simulink library "lib_Sensors"  (R2017b)
settings: Solver=VariableStepAuto  StartTime=0.0  StopTime=10.0  RelTol=1e-3
settings Model: Creator=Di Russo  LastModifiedBy=Vraj M
settings CodeAppCC: StateflowObjectComments=on

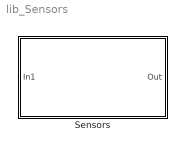
== system lib_Sensors ==
  Sensors : Subsystem

== system lib_Sensors/Sensors ==
  In1 : Inport
  Analog : Subsystem
  Bus Creator : BusCreator  Inputs=3
  Bus Selector : BusSelector  OutputSignals=CAN
  CAN : Subsystem
  Digital : Subsystem
  Out : Outport
  wires:
  Digital/1(Out1) -> Bus Creator/3  "from_Digital"
  Analog/1(Out1) -> Bus Creator/2  "from_Analog"
  CAN/1(Out1) -> Bus Creator/1  "from_CAN"
  Bus Selector/1 -> CAN/1(In1)  "<CAN>"
  In1/1 -> Bus Selector/1, Analog/1(In1), Digital/1(In1)
  Bus Creator/1 -> Out/1

== system lib_Sensors/Sensors/Analog ==
  In1 : Inport
  Bus Creator : BusCreator  Inputs=4
  Bus Selector : BusSelector  OutputSignals=Driver_Signals.drv_APP1,Driver_Signals.drv_APP2,DC_mode,Driver_Signals.Sport_Mode_SW
  Data Type Conversion : DataTypeConversion
  Data Type Conversion1 : DataTypeConversion
  Data Type Conversion2 : DataTypeConversion
  Out1 : Outport
  wires:
  Bus Selector/4 -> Bus Creator/4  "<Sport_Mode_SW>"
  Bus Selector/1 -> Data Type Conversion2/1  "<drv_APP1>"
  Bus Selector/2 -> Data Type Conversion1/1  "<drv_APP2>"
  Bus Selector/3 -> Data Type Conversion/1  "<DC_mode>"
  Bus Creator/1 -> Out1/1
  In1/1 -> Bus Selector/1
  Data Type Conversion2/1 -> Bus Creator/1  "Driver_APP1"
  Data Type Conversion1/1 -> Bus Creator/2  "Driver_APP2"
  Data Type Conversion/1 -> Bus Creator/3  "DC_mode"

== system lib_Sensors/Sensors/CAN ==
  In1 : Inport
  Bus Creator : BusCreator  Inputs=3
  EBCAN : Subsystem
  HV_CAN : Subsystem
  VEH_CAN : Subsystem
  Out1 : Outport
  wires:
  VEH_CAN/1(Out1) -> Bus Creator/1  "fromVEH_CAN"
  Bus Creator/1 -> Out1/1  "from_CAN"
  EBCAN/1(Out1) -> Bus Creator/2  "fromEBCAN"
  HV_CAN/1(Out1) -> Bus Creator/3  "fromHV_CAN"
  In1/1 -> HV_CAN/1(In1), EBCAN/1(In1), VEH_CAN/1(In1)

== system lib_Sensors/Sensors/Digital ==
  In1 : Inport
  Bus Creator : BusCreator  Inputs=3
  Bus Selector : BusSelector  OutputSignals=Driver_Signals.SW_Regen_Disable,Driver_Signals.SW_Engine_ON,Driver_Signals.SW_CS_ON
  Data Type Conversion : DataTypeConversion
  Data Type Conversion1 : DataTypeConversion
  Data Type Conversion2 : DataTypeConversion
  Out1 : Outport
  wires:
  Bus Creator/1 -> Out1/1  "Digital"
  Data Type Conversion1/1 -> Bus Creator/1  "SW_Regen_Disable"
  Data Type Conversion2/1 -> Bus Creator/3  "SW_CS_ON"
  Data Type Conversion/1 -> Bus Creator/2  "SW_Engine_ON"
  Bus Selector/3 -> Data Type Conversion2/1  "<SW_CS_ON>"
  Bus Selector/2 -> Data Type Conversion/1  "<SW_Engine_ON>"
  Bus Selector/1 -> Data Type Conversion1/1  "<SW_Regen_Disable>"
  In1/1 -> Bus Selector/1

== system lib_Sensors/Sensors/CAN/EBCAN ==
  In1 : Inport
  BMS_Antrieb : Subsystem
  Bus Creator : BusCreator  Inputs=3
  Bus Selector : BusSelector  OutputSignals=ECM_CAN,BMS_CAN.BMS_Hybrid
  CCM : Subsystem
  ECM : Subsystem
  Out1 : Outport
  wires:
  ECM/1(Out1) -> Bus Creator/1  "from_ECM"
  BMS_Antrieb/1(Out1) -> Bus Creator/2  "from_BMSAntrieb"
  Bus Creator/1 -> Out1/1
  CCM/1(Out1) -> Bus Creator/3  "from_CCM"
  In1/1 -> Bus Selector/1
  Bus Selector/1 -> ECM/1(In1)  "<ECM_CAN>"
  Bus Selector/2 -> CCM/1(In1), BMS_Antrieb/1(In1)  "<BMS_Hybrid>"

== system lib_Sensors/Sensors/CAN/HV_CAN ==
  In1 : Inport
  BMS_Hybrid : Subsystem
  Bus Creator : BusCreator  Inputs=4
  Bus Selector : BusSelector  OutputSignals=MCU_CAN,BMS_CAN.BMS_Plugin,OBC_CAN
  Clutch : Subsystem
  MCU : Subsystem
  OBC : Subsystem
  Out1 : Outport
  wires:
  MCU/1(Out1) -> Bus Creator/2  "from_MCU"
  BMS_Hybrid/1(Out1) -> Bus Creator/3  "from_BMSHybrid"
  OBC/1(Out1) -> Bus Creator/4  "from_OBC"
  Bus Creator/1 -> Out1/1
  In1/1 -> Bus Selector/1
  Bus Selector/1 -> Clutch/1(In1), MCU/1(In1)  "<MCU_CAN>"
  Bus Selector/2 -> BMS_Hybrid/1(In1)  "<BMS_Plugin>"
  Bus Selector/3 -> OBC/1(In1)  "<OBC_CAN>"
  Clutch/1(Out1) -> Bus Creator/1

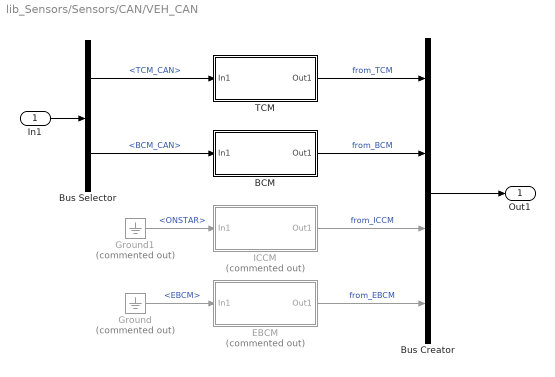
== system lib_Sensors/Sensors/CAN/VEH_CAN ==
  In1 : Inport
  BCM : Subsystem
  Bus Creator : BusCreator  Inputs=4
  Bus Selector : BusSelector  OutputSignals=TCM_CAN,BCM_CAN
  EBCM : Subsystem  Commented=on
  Ground : Ground  Commented=on
  Ground1 : Ground  Commented=on
  ICCM : Subsystem  Commented=on
  TCM : Subsystem
  Out1 : Outport
  wires:
  In1/1 -> Bus Selector/1
  TCM/1(Out1) -> Bus Creator/1  "from_TCM"
  BCM/1(Out1) -> Bus Creator/2  "from_BCM"
  ICCM/1(Out1) -> Bus Creator/3  "from_ICCM"
  EBCM/1(Out1) -> Bus Creator/4  "from_EBCM"
  Bus Creator/1 -> Out1/1
  Bus Selector/1 -> TCM/1(In1)  "<TCM_CAN>"
  Bus Selector/2 -> BCM/1(In1)  "<BCM_CAN>"
  Ground1/1 -> ICCM/1(In1)  "<ONSTAR>"
  Ground/1 -> EBCM/1(In1)  "<EBCM>"

== system lib_Sensors/Sensors/CAN/EBCAN/BMS_Antrieb ==
  In1 : Inport
  Bus Creator : BusCreator  Inputs=2
  Bus Selector : BusSelector  OutputSignals=NMH_BMS,ISO_Hybrid_01_Resp
  ISO_Hybrid_01_Resp : Subsystem
  NMH_BMS : Subsystem
  Out1 : Outport
  wires:
  In1/1 -> Bus Selector/1
  Bus Selector/1 -> NMH_BMS/1(In1)  "<NMH_BMS>"
  NMH_BMS/1(Out1) -> Bus Creator/1
  ISO_Hybrid_01_Resp/1(Out1) -> Bus Creator/2
  Bus Creator/1 -> Out1/1
  Bus Selector/2 -> ISO_Hybrid_01_Resp/1(In1)  "<ISO_Hybrid_01_Resp>"

== system lib_Sensors/Sensors/CAN/EBCAN/CCM ==
  In1 : Inport
  Bus Creator : BusCreator  Inputs=2
  Bus Selector : BusSelector  OutputSignals=NMH_BMS,ISO_Hybrid_01_Resp
  ISO_Hybrid_01_Resp : Subsystem
  NMH_BMS : Subsystem
  Out1 : Outport
  wires:
  Bus Selector/2 -> ISO_Hybrid_01_Resp/1(In1)  "<ISO_Hybrid_01_Resp>"
  Bus Creator/1 -> Out1/1
  ISO_Hybrid_01_Resp/1(Out1) -> Bus Creator/2
  NMH_BMS/1(Out1) -> Bus Creator/1
  Bus Selector/1 -> NMH_BMS/1(In1)  "<NMH_BMS>"
  In1/1 -> Bus Selector/1

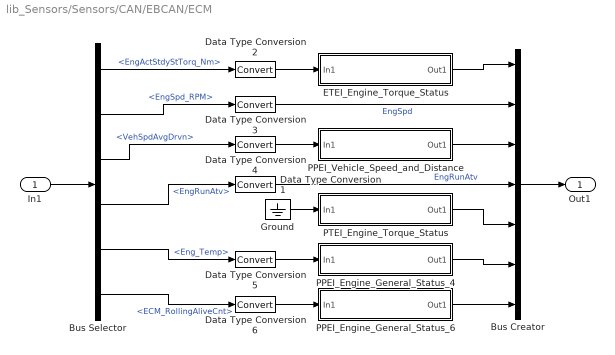
== system lib_Sensors/Sensors/CAN/EBCAN/ECM ==
  In1 : Inport
  Bus Creator : BusCreator  Inputs=7
  Bus Selector : BusSelector  OutputSignals=Sensors_to_ECM.EngActStdyStTorq_Nm,Sensors_to_ECM.EngSpd_RPM,ECM_to_Actuators.VehSpdAvgDrvn,ECM_to_Actuators.EngRunAtv,ECM_to_Actuators.Eng_Temp,ECM_to_Actuators.ECM_RollingAliveCnt
  Data Type Conversion{1..6} (6 alike) : DataTypeConversion
  ETEI_Engine_Torque_Status : Subsystem
  Ground : Ground
  PPEI_Engine_General_Status_4 : Subsystem
  PPEI_Engine_General_Status_6 : Subsystem
  PPEI_Vehicle_Speed_and_Distance : Subsystem
  PTEI_Engine_Torque_Status : Subsystem
  Out1 : Outport
  wires:
  Bus Selector/6 -> Data Type Conversion6/1  "<ECM_RollingAliveCnt>"
  Bus Selector/5 -> Data Type Conversion5/1  "<Eng_Temp>"
  Bus Selector/3 -> Data Type Conversion4/1  "<VehSpdAvgDrvn>"
  Bus Selector/1 -> Data Type Conversion2/1  "<EngActStdyStTorq_Nm>"
  In1/1 -> Bus Selector/1
  Data Type Conversion2/1 -> ETEI_Engine_Torque_Status/1(In1)
  Bus Selector/2 -> Data Type Conversion3/1  "<EngSpd_RPM>"
  Data Type Conversion4/1 -> PPEI_Vehicle_Speed_and_Distance/1(In1)
  ETEI_Engine_Torque_Status/1(Out1) -> Bus Creator/1
  PPEI_Vehicle_Speed_and_Distance/1(Out1) -> Bus Creator/3
  Bus Creator/1 -> Out1/1
  Bus Selector/4 -> Data Type Conversion1/1  "<EngRunAtv>"
  Ground/1 -> PTEI_Engine_Torque_Status/1(In1)
  PTEI_Engine_Torque_Status/1(Out1) -> Bus Creator/5
  Data Type Conversion5/1 -> PPEI_Engine_General_Status_4/1(In1)
  PPEI_Engine_General_Status_4/1(Out1) -> Bus Creator/6
  Data Type Conversion6/1 -> PPEI_Engine_General_Status_6/1(In1)
  PPEI_Engine_General_Status_6/1(Out1) -> Bus Creator/7
  Data Type Conversion3/1 -> Bus Creator/2  "EngSpd"
  Data Type Conversion1/1 -> Bus Creator/4  "EngRunAtv"

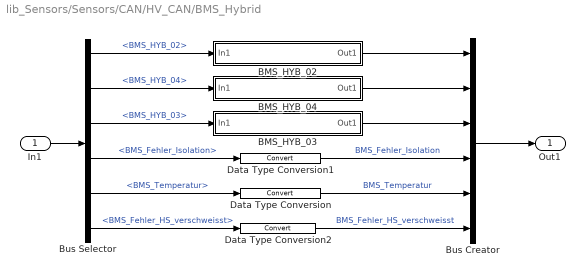
== system lib_Sensors/Sensors/CAN/HV_CAN/BMS_Hybrid ==
  In1 : Inport
  BMS_HYB_02 : Subsystem
  BMS_HYB_03 : Subsystem
  BMS_HYB_04 : Subsystem
  Bus Creator : BusCreator  Inputs=6
  Bus Selector : BusSelector  OutputSignals=BMS_HYB_02,BMS_HYB_04,BMS_HYB_03,BMS_HYB_02.BMS_Fehler_Isolation,BMS_HYB_06.BMS_Temperatur,BMS_HYB_02.BMS_Fehler_HS_verschweisst
  Data Type Conversion : DataTypeConversion
  Data Type Conversion1 : DataTypeConversion
  Data Type Conversion2 : DataTypeConversion
  Out1 : Outport
  wires:
  Bus Selector/6 -> Data Type Conversion2/1  "<BMS_Fehler_HS_verschweisst>"
  Data Type Conversion1/1 -> Bus Creator/4  "BMS_Fehler_Isolation"
  Data Type Conversion/1 -> Bus Creator/5  "BMS_Temperatur"
  In1/1 -> Bus Selector/1
  Bus Selector/1 -> BMS_HYB_02/1(In1)  "<BMS_HYB_02>"
  Bus Selector/2 -> BMS_HYB_04/1(In1)  "<BMS_HYB_04>"
  Bus Creator/1 -> Out1/1
  BMS_HYB_02/1(Out1) -> Bus Creator/1
  BMS_HYB_04/1(Out1) -> Bus Creator/2
  Bus Selector/3 -> BMS_HYB_03/1(In1)  "<BMS_HYB_03>"
  BMS_HYB_03/1(Out1) -> Bus Creator/3
  Bus Selector/4 -> Data Type Conversion1/1  "<BMS_Fehler_Isolation>"
  Bus Selector/5 -> Data Type Conversion/1  "<BMS_Temperatur>"
  Data Type Conversion2/1 -> Bus Creator/6  "BMS_Fehler_HS_verschweisst"

== system lib_Sensors/Sensors/CAN/HV_CAN/Clutch ==
  In1 : Inport
  Bus Creator : BusCreator  Inputs=2
  Bus Selector : BusSelector  OutputSignals=MCU_to _Actuator.EngageClutch,Sensors_to_MCU.clt_plant_spd_in
  Data Type Conversion : DataTypeConversion
  Data Type Conversion1 : DataTypeConversion
  Out1 : Outport
  wires:
  Bus Selector/2 -> Data Type Conversion1/1  "<clt_plant_spd_in>"
  Data Type Conversion1/1 -> Bus Creator/2  "CY01_AngSpdCurr"
  Data Type Conversion/1 -> Bus Creator/1  "CY01_posCurr"
  Bus Selector/1 -> Data Type Conversion/1  "<EngageClutch>"
  Bus Creator/1 -> Out1/1  "Clutch"
  In1/1 -> Bus Selector/1

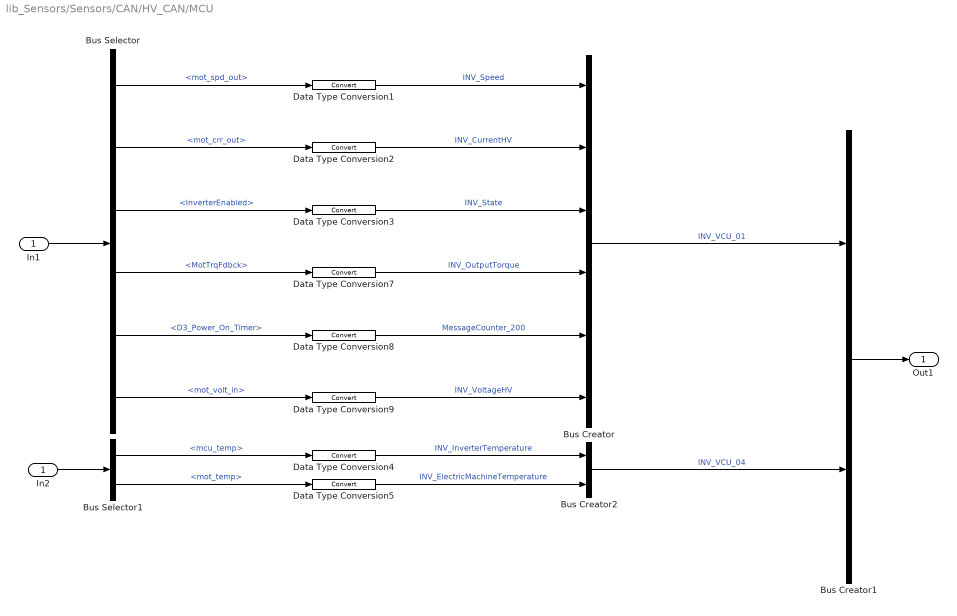
== system lib_Sensors/Sensors/CAN/HV_CAN/MCU ==
  In1 : Inport
  Bus Creator : BusCreator  Inputs=6
  Bus Creator1 : BusCreator  Inputs=2
  Bus Creator2 : BusCreator  Inputs=2
  Bus Selector : BusSelector  OutputSignals=Sensors_to_MCU.mot_spd_out,Sensors_to_MCU.mot_crr_out,MCU_to _Actuator.InverterEnabled,MCU_to _Actuator.MotTrqFdbck,MCU_to _Actuator.D3_Power_On_Timer,Sensors_to_MCU.mot_volt_in
  Bus Selector1 : BusSelector  OutputSignals=Sensors_to_MCU.mcu_temp,Sensors_to_MCU.mot_temp
  Data Type Conversion{1..5,7..9} (8 alike) : DataTypeConversion
  In2 : InportShadow
  Out1 : Outport
  wires:
  Bus Creator1/1 -> Out1/1
  Bus Creator2/1 -> Bus Creator1/2  "INV_VCU_04"
  In2/1 -> Bus Selector1/1
  Bus Selector1/1 -> Data Type Conversion4/1  "<mcu_temp>"
  Data Type Conversion5/1 -> Bus Creator2/2  "INV_ElectricMachineTemperature"
  Bus Selector1/2 -> Data Type Conversion5/1  "<mot_temp>"
  Data Type Conversion4/1 -> Bus Creator2/1  "INV_InverterTemperature"
  Data Type Conversion9/1 -> Bus Creator/6  "INV_VoltageHV"
  Data Type Conversion8/1 -> Bus Creator/5  "MessageCounter_200"
  Data Type Conversion7/1 -> Bus Creator/4  "INV_OutputTorque"
  Bus Selector/1 -> Data Type Conversion1/1  "<mot_spd_out>"
  Bus Selector/2 -> Data Type Conversion2/1  "<mot_crr_out>"
  Bus Selector/3 -> Data Type Conversion3/1  "<InverterEnabled>"
  Data Type Conversion1/1 -> Bus Creator/1  "INV_Speed"
  Data Type Conversion2/1 -> Bus Creator/2  "INV_CurrentHV"
  Data Type Conversion3/1 -> Bus Creator/3  "INV_State"
  Bus Creator/1 -> Bus Creator1/1  "INV_VCU_01"
  Bus Selector/5 -> Data Type Conversion8/1  "<D3_Power_On_Timer>"
  Bus Selector/4 -> Data Type Conversion7/1  "<MotTrqFdbck>"
  Bus Selector/6 -> Data Type Conversion9/1  "<mot_volt_in>"
  In1/1 -> Bus Selector/1

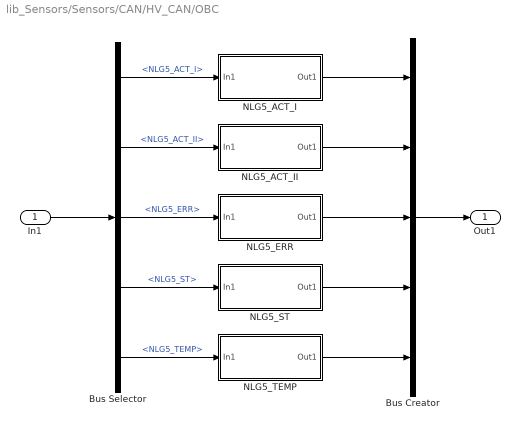
== system lib_Sensors/Sensors/CAN/HV_CAN/OBC ==
  In1 : Inport
  Bus Creator : BusCreator  Inputs=5
  Bus Selector : BusSelector  OutputSignals=NLG5_ACT_I,NLG5_ACT_II,NLG5_ERR,NLG5_ST,NLG5_TEMP
  NLG5_ACT_I : Subsystem
  NLG5_ACT_II : Subsystem
  NLG5_ERR : Subsystem
  NLG5_ST : Subsystem
  NLG5_TEMP : Subsystem
  Out1 : Outport
  wires:
  Bus Creator/1 -> Out1/1
  NLG5_TEMP/1(Out1) -> Bus Creator/5
  Bus Selector/5 -> NLG5_TEMP/1(In1)  "<NLG5_TEMP>"
  NLG5_ST/1(Out1) -> Bus Creator/4
  Bus Selector/4 -> NLG5_ST/1(In1)  "<NLG5_ST>"
  Bus Selector/3 -> NLG5_ERR/1(In1)  "<NLG5_ERR>"
  NLG5_ERR/1(Out1) -> Bus Creator/3
  NLG5_ACT_II/1(Out1) -> Bus Creator/2
  Bus Selector/2 -> NLG5_ACT_II/1(In1)  "<NLG5_ACT_II>"
  NLG5_ACT_I/1(Out1) -> Bus Creator/1
  Bus Selector/1 -> NLG5_ACT_I/1(In1)  "<NLG5_ACT_I>"
  In1/1 -> Bus Selector/1

== system lib_Sensors/Sensors/CAN/VEH_CAN/BCM ==
  In1 : Inport
  Bus Creator : BusCreator  Inputs=2
  Bus Selector : BusSelector  OutputSignals=SysPwrMd,BrkPdlPos
  Data Type Conversion : DataTypeConversion
  Data Type Conversion1 : DataTypeConversion
  PPEI_Brake_Apply_Status : Subsystem
  PPEI_Platfrom_General_Status : Subsystem
  Out1 : Outport
  wires:
  In1/1 -> Bus Selector/1
  Bus Selector/1 -> Data Type Conversion/1  "<SysPwrMd>"
  Bus Selector/2 -> Data Type Conversion1/1  "<BrkPdlPos>"
  PPEI_Platfrom_General_Status/1(Out1) -> Bus Creator/1
  PPEI_Brake_Apply_Status/1(Out1) -> Bus Creator/2
  Bus Creator/1 -> Out1/1
  Data Type Conversion/1 -> PPEI_Platfrom_General_Status/1(In1)
  Data Type Conversion1/1 -> PPEI_Brake_Apply_Status/1(In1)

== system lib_Sensors/Sensors/CAN/VEH_CAN/EBCM ==
  In1 : Inport
  Bus Selector : BusSelector  OutputSignals=PPEI_Chassis_General_Status_1.BrkPdlDrvAppPrsDetcd
  Constant : Constant  OutDataTypeStr=boolean
  PPEI_Chassis_General_Status_1 : Subsystem
  Terminator : Terminator
  Out1 : Outport
  wires:
  Bus Selector/1 -> Terminator/1  "<BrkPdlDrvAppPrsDetcd>"
  PPEI_Chassis_General_Status_1/1(Out1) -> Out1/1
  In1/1 -> Bus Selector/1
  Constant/1 -> PPEI_Chassis_General_Status_1/1(In1)

== system lib_Sensors/Sensors/CAN/VEH_CAN/ICCM ==
  In1 : Inport
  Out1 : Outport
  wires:
  In1/1 -> Out1/1

== system lib_Sensors/Sensors/CAN/VEH_CAN/TCM ==
  In1 : Inport
  Bus Creator : BusCreator  Inputs=4
  Bus Selector : BusSelector  OutputSignals=TCM_to _Actuator.TransEstGear,TCM_to _Actuator.LockupCmd,TCM_to _Actuator.TrnsShftLvrPos,Sensors_to_TCM.gb_trq_ratio
  Data Type Conversion{,1..3} (4 alike) : DataTypeConversion
  Out1 : Outport
  wires:
  Bus Selector/4 -> Data Type Conversion3/1  "<gb_trq_ratio>"
  Bus Selector/3 -> Data Type Conversion2/1  "<TrnsShftLvrPos>"
  Bus Selector/2 -> Data Type Conversion1/1  "<LockupCmd>"
  Bus Selector/1 -> Data Type Conversion/1  "<TransEstGear>"
  Data Type Conversion3/1 -> Bus Creator/4  "TrnGrRat"
  Data Type Conversion2/1 -> Bus Creator/3  "TrnsShftLvrPos"
  Data Type Conversion1/1 -> Bus Creator/2  "TrnsTrqCnvCltCmndMd"
  In1/1 -> Bus Selector/1
  Bus Creator/1 -> Out1/1
  Data Type Conversion/1 -> Bus Creator/1  "TransEstGear"

== system lib_Sensors/Sensors/CAN/EBCAN/BMS_Antrieb/ISO_Hybrid_01_Resp ==
  In1 : Inport
  Bus Creator : BusCreator  Inputs=3
  Bus Selector : BusSelector  OutputSignals=ISO_Hybrid_01_Resp_Data_4,ISO_Hybrid_01_Resp_Data_5,ISO_Hybrid_01_Resp_Data_6
  Data Type Conversion : DataTypeConversion
  Data Type Conversion1 : DataTypeConversion
  Data Type Conversion2 : DataTypeConversion
  Out1 : Outport
  wires:
  Data Type Conversion2/1 -> Bus Creator/3  "ISO_Hybrid_01_Resp_Data_byte_5"
  Data Type Conversion1/1 -> Bus Creator/2  "ISO_Hybrid_01_Resp_Data_byte_4"
  Data Type Conversion/1 -> Bus Creator/1  "ISO_Hybrid_01_Resp_Data_byte_3"
  Bus Creator/1 -> Out1/1  "ISO_Hybrid_01_Resp_Data"
  Bus Selector/3 -> Data Type Conversion2/1  "<ISO_Hybrid_01_Resp_Data_6>"
  Bus Selector/2 -> Data Type Conversion1/1  "<ISO_Hybrid_01_Resp_Data_5>"
  Bus Selector/1 -> Data Type Conversion/1  "<ISO_Hybrid_01_Resp_Data_4>"
  In1/1 -> Bus Selector/1

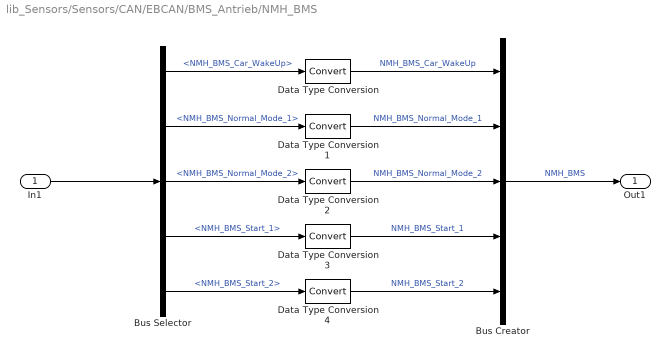
== system lib_Sensors/Sensors/CAN/EBCAN/BMS_Antrieb/NMH_BMS ==
  In1 : Inport
  Bus Creator : BusCreator  Inputs=5
  Bus Selector : BusSelector  OutputSignals=NMH_BMS_Car_WakeUp,NMH_BMS_Normal_Mode_1,NMH_BMS_Normal_Mode_2,NMH_BMS_Start_1,NMH_BMS_Start_2
  Data Type Conversion{,1..4} (5 alike) : DataTypeConversion
  Out1 : Outport
  wires:
  Data Type Conversion4/1 -> Bus Creator/5  "NMH_BMS_Start_2"
  Data Type Conversion3/1 -> Bus Creator/4  "NMH_BMS_Start_1"
  Data Type Conversion2/1 -> Bus Creator/3  "NMH_BMS_Normal_Mode_2"
  Data Type Conversion1/1 -> Bus Creator/2  "NMH_BMS_Normal_Mode_1"
  Data Type Conversion/1 -> Bus Creator/1  "NMH_BMS_Car_WakeUp"
  Bus Selector/1 -> Data Type Conversion/1  "<NMH_BMS_Car_WakeUp>"
  Bus Selector/2 -> Data Type Conversion1/1  "<NMH_BMS_Normal_Mode_1>"
  Bus Selector/3 -> Data Type Conversion2/1  "<NMH_BMS_Normal_Mode_2>"
  Bus Selector/4 -> Data Type Conversion3/1  "<NMH_BMS_Start_1>"
  Bus Selector/5 -> Data Type Conversion4/1  "<NMH_BMS_Start_2>"
  Bus Creator/1 -> Out1/1  "NMH_BMS"
  In1/1 -> Bus Selector/1

== system lib_Sensors/Sensors/CAN/EBCAN/CCM/ISO_Hybrid_01_Resp ==
  In1 : Inport
  Bus Creator : BusCreator  Inputs=3
  Bus Selector : BusSelector  OutputSignals=ISO_Hybrid_01_Resp_Data_4,ISO_Hybrid_01_Resp_Data_5,ISO_Hybrid_01_Resp_Data_6
  Data Type Conversion : DataTypeConversion
  Data Type Conversion1 : DataTypeConversion
  Data Type Conversion2 : DataTypeConversion
  Out1 : Outport
  wires:
  In1/1 -> Bus Selector/1
  Bus Selector/1 -> Data Type Conversion/1  "<ISO_Hybrid_01_Resp_Data_4>"
  Bus Selector/2 -> Data Type Conversion1/1  "<ISO_Hybrid_01_Resp_Data_5>"
  Bus Selector/3 -> Data Type Conversion2/1  "<ISO_Hybrid_01_Resp_Data_6>"
  Bus Creator/1 -> Out1/1  "ISO_Hybrid_01_Resp_Data"
  Data Type Conversion/1 -> Bus Creator/1  "ISO_Hybrid_01_Resp_Data_byte_3"
  Data Type Conversion1/1 -> Bus Creator/2  "ISO_Hybrid_01_Resp_Data_byte_4"
  Data Type Conversion2/1 -> Bus Creator/3  "ISO_Hybrid_01_Resp_Data_byte_5"

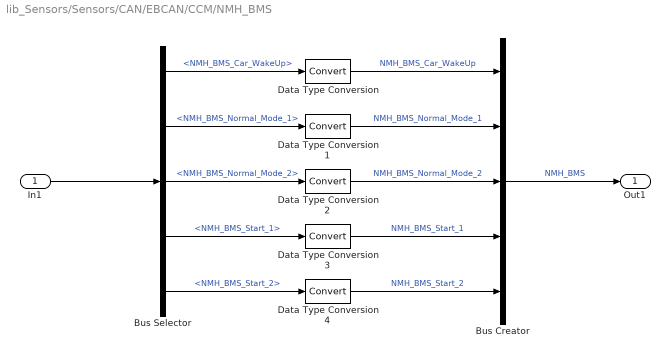
== system lib_Sensors/Sensors/CAN/EBCAN/CCM/NMH_BMS ==
  In1 : Inport
  Bus Creator : BusCreator  Inputs=5
  Bus Selector : BusSelector  OutputSignals=NMH_BMS_Car_WakeUp,NMH_BMS_Normal_Mode_1,NMH_BMS_Normal_Mode_2,NMH_BMS_Start_1,NMH_BMS_Start_2
  Data Type Conversion{,1..4} (5 alike) : DataTypeConversion
  Out1 : Outport
  wires:
  In1/1 -> Bus Selector/1
  Bus Creator/1 -> Out1/1  "NMH_BMS"
  Bus Selector/5 -> Data Type Conversion4/1  "<NMH_BMS_Start_2>"
  Bus Selector/4 -> Data Type Conversion3/1  "<NMH_BMS_Start_1>"
  Bus Selector/3 -> Data Type Conversion2/1  "<NMH_BMS_Normal_Mode_2>"
  Bus Selector/2 -> Data Type Conversion1/1  "<NMH_BMS_Normal_Mode_1>"
  Bus Selector/1 -> Data Type Conversion/1  "<NMH_BMS_Car_WakeUp>"
  Data Type Conversion/1 -> Bus Creator/1  "NMH_BMS_Car_WakeUp"
  Data Type Conversion1/1 -> Bus Creator/2  "NMH_BMS_Normal_Mode_1"
  Data Type Conversion2/1 -> Bus Creator/3  "NMH_BMS_Normal_Mode_2"
  Data Type Conversion3/1 -> Bus Creator/4  "NMH_BMS_Start_1"
  Data Type Conversion4/1 -> Bus Creator/5  "NMH_BMS_Start_2"

== system lib_Sensors/Sensors/CAN/EBCAN/ECM/ETEI_Engine_Torque_Status ==
  In1 : Inport
  Out1 : Outport
  wires:
  In1/1 -> Out1/1  "EngActStdyStTorq"

== system lib_Sensors/Sensors/CAN/EBCAN/ECM/PPEI_Engine_General_Status_4 ==
  In1 : Inport
  Out1 : Outport
  wires:
  In1/1 -> Out1/1  "EngCltTmp"

== system lib_Sensors/Sensors/CAN/EBCAN/ECM/PPEI_Engine_General_Status_6 ==
  In1 : Inport
  Out1 : Outport
  wires:
  In1/1 -> Out1/1  "PlatEngSpdCmdStARC"

== system lib_Sensors/Sensors/CAN/EBCAN/ECM/PPEI_Vehicle_Speed_and_Distance ==
  In1 : Inport
  Out1 : Outport
  wires:
  In1/1 -> Out1/1  "VehSpdAvgDrvn"

== system lib_Sensors/Sensors/CAN/EBCAN/ECM/PTEI_Engine_Torque_Status ==
  In1 : Inport
  Out1 : Outport
  wires:
  In1/1 -> Out1/1  "CrksftNTrnsRegCmdTq"

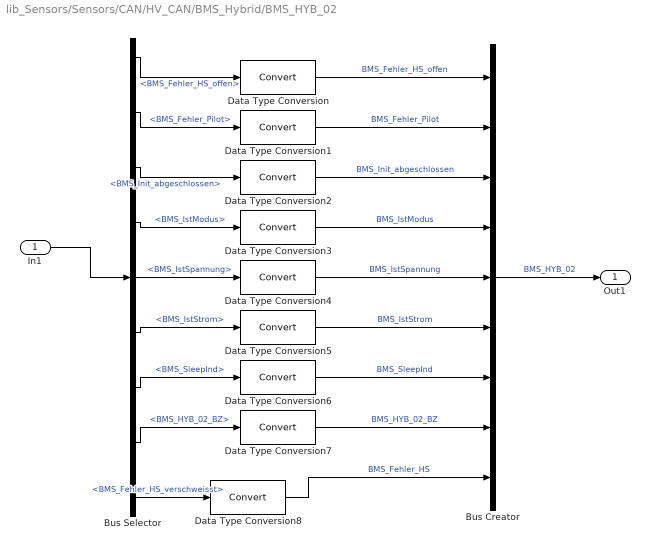
== system lib_Sensors/Sensors/CAN/HV_CAN/BMS_Hybrid/BMS_HYB_02 ==
  In1 : Inport
  Bus Creator : BusCreator  Inputs=9
  Bus Selector : BusSelector  OutputSignals=BMS_Fehler_HS_offen,BMS_Fehler_Pilot,BMS_Init_abgeschlossen,BMS_IstModus,BMS_IstSpannung,BMS_IstStrom,BMS_SleepInd,BMS_HYB_02_BZ,BMS_Fehler_HS_verschweisst
  Data Type Conversion{,1..8} (9 alike) : DataTypeConversion
  Out1 : Outport
  wires:
  Data Type Conversion8/1 -> Bus Creator/9  "BMS_Fehler_HS"
  Data Type Conversion7/1 -> Bus Creator/8  "BMS_HYB_02_BZ"
  Data Type Conversion6/1 -> Bus Creator/7  "BMS_SleepInd"
  Data Type Conversion5/1 -> Bus Creator/6  "BMS_IstStrom"
  Data Type Conversion4/1 -> Bus Creator/5  "BMS_IstSpannung"
  Data Type Conversion3/1 -> Bus Creator/4  "BMS_IstModus"
  Data Type Conversion2/1 -> Bus Creator/3  "BMS_Init_abgeschlossen"
  Data Type Conversion1/1 -> Bus Creator/2  "BMS_Fehler_Pilot"
  Data Type Conversion/1 -> Bus Creator/1  "BMS_Fehler_HS_offen"
  Bus Selector/1 -> Data Type Conversion/1  "<BMS_Fehler_HS_offen>"
  Bus Selector/2 -> Data Type Conversion1/1  "<BMS_Fehler_Pilot>"
  Bus Selector/3 -> Data Type Conversion2/1  "<BMS_Init_abgeschlossen>"
  Bus Selector/4 -> Data Type Conversion3/1  "<BMS_IstModus>"
  Bus Selector/5 -> Data Type Conversion4/1  "<BMS_IstSpannung>"
  Bus Selector/6 -> Data Type Conversion5/1  "<BMS_IstStrom>"
  Bus Selector/7 -> Data Type Conversion6/1  "<BMS_SleepInd>"
  Bus Creator/1 -> Out1/1  "BMS_HYB_02"
  In1/1 -> Bus Selector/1
  Bus Selector/8 -> Data Type Conversion7/1  "<BMS_HYB_02_BZ>"
  Bus Selector/9 -> Data Type Conversion8/1  "<BMS_Fehler_HS_verschweisst>"

== system lib_Sensors/Sensors/CAN/HV_CAN/BMS_Hybrid/BMS_HYB_03 ==
  In1 : Inport
  Bus Selector : BusSelector  OutputSignals=BMS_SOC
  Data Type Conversion : DataTypeConversion
  Out1 : Outport
  wires:
  Data Type Conversion/1 -> Out1/1  "BMS_SOC"
  Bus Selector/1 -> Data Type Conversion/1  "<BMS_SOC>"
  In1/1 -> Bus Selector/1

== system lib_Sensors/Sensors/CAN/HV_CAN/BMS_Hybrid/BMS_HYB_04 ==
  In1 : Inport
  Bus Selector : BusSelector  OutputSignals=BMS_Spannung_ZwKr
  Data Type Conversion : DataTypeConversion
  Out1 : Outport
  wires:
  Data Type Conversion/1 -> Out1/1  "BMS_Spannung_ZwKr"
  In1/1 -> Bus Selector/1  "BMS_Spannung_ZwKr"
  Bus Selector/1 -> Data Type Conversion/1  "<BMS_Spannung_ZwKr>"

== system lib_Sensors/Sensors/CAN/HV_CAN/OBC/NLG5_ACT_I ==
  In1 : Inport
  Bus Creator : BusCreator  Inputs=4
  Bus Selector : BusSelector  OutputSignals=signal1,NLG5_MV_ACT,NLG5_OV_ACT,NLG5_OC_ACT
  Data Type Conversion{,1..3} (4 alike) : DataTypeConversion
  Out1 : Outport
  wires:
  Bus Creator/1 -> Out1/1  "NLG5_ACT_I"
  Data Type Conversion3/1 -> Bus Creator/4  "NLG5_OC_ACT"
  Data Type Conversion2/1 -> Bus Creator/3  "NLG5_OV_ACT"
  Data Type Conversion1/1 -> Bus Creator/2  "NLG5_MV_ACT"
  Data Type Conversion/1 -> Bus Creator/1  "NLG5_MC_ACT"
  Bus Selector/4 -> Data Type Conversion3/1  "<NLG5_OC_ACT>"
  Bus Selector/3 -> Data Type Conversion2/1  "<NLG5_OV_ACT>"
  Bus Selector/2 -> Data Type Conversion1/1  "<NLG5_MV_ACT>"
  Bus Selector/1 -> Data Type Conversion/1  "<signal1>"
  In1/1 -> Bus Selector/1

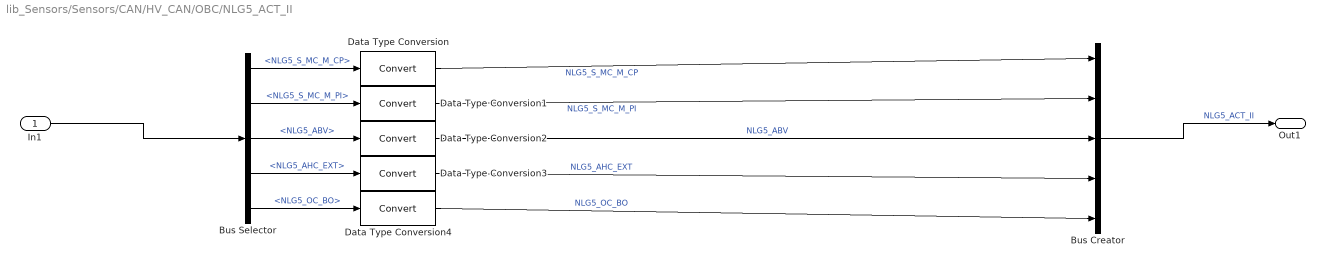
== system lib_Sensors/Sensors/CAN/HV_CAN/OBC/NLG5_ACT_II ==
  In1 : Inport
  Bus Creator : BusCreator  Inputs=5
  Bus Selector : BusSelector  OutputSignals=NLG5_S_MC_M_CP,NLG5_S_MC_M_PI,NLG5_ABV,NLG5_AHC_EXT,NLG5_OC_BO
  Data Type Conversion{,1..4} (5 alike) : DataTypeConversion
  Out1 : Outport
  wires:
  Data Type Conversion4/1 -> Bus Creator/5  "NLG5_OC_BO"
  Bus Selector/5 -> Data Type Conversion4/1  "<NLG5_OC_BO>"
  In1/1 -> Bus Selector/1
  Bus Selector/1 -> Data Type Conversion/1  "<NLG5_S_MC_M_CP>"
  Bus Selector/2 -> Data Type Conversion1/1  "<NLG5_S_MC_M_PI>"
  Bus Selector/3 -> Data Type Conversion2/1  "<NLG5_ABV>"
  Bus Selector/4 -> Data Type Conversion3/1  "<NLG5_AHC_EXT>"
  Data Type Conversion/1 -> Bus Creator/1  "NLG5_S_MC_M_CP"
  Data Type Conversion1/1 -> Bus Creator/2  "NLG5_S_MC_M_PI"
  Data Type Conversion2/1 -> Bus Creator/3  "NLG5_ABV"
  Data Type Conversion3/1 -> Bus Creator/4  "NLG5_AHC_EXT"
  Bus Creator/1 -> Out1/1  "NLG5_ACT_II"

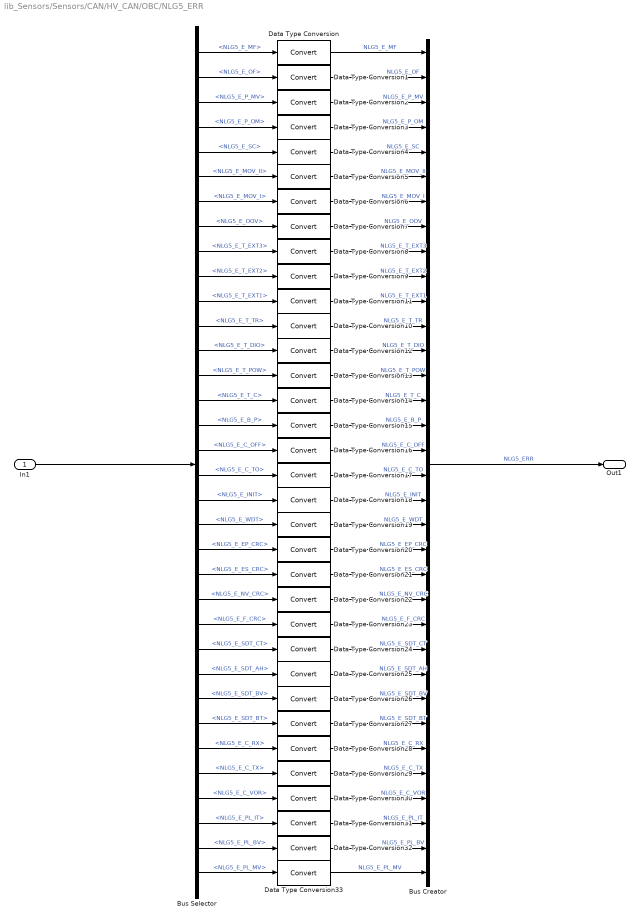
== system lib_Sensors/Sensors/CAN/HV_CAN/OBC/NLG5_ERR ==
  In1 : Inport
  Bus Creator : BusCreator  Inputs=34
  Bus Selector : BusSelector  OutputSignals=NLG5_E_MF,NLG5_E_OF,NLG5_E_P_MV,NLG5_E_P_OM,NLG5_E_SC,NLG5_E_MOV_II,NLG5_E_MOV_I,NLG5_E_OOV,NLG5_E_T_EXT3,NLG5_E_T_EXT2,NLG5_E_T_EXT1,NLG5_E_T_TR,NLG5_E_T_DIO,NLG5_E_T_POW,NLG5_E_T_C,NLG5_E_B_P,NLG5_E_C_OFF,NLG5_E_C_TO,NLG5_E_INIT,NLG5_E_WDT,NLG5_E_EP_CRC,NLG5_E_ES_CRC,NLG5_E_NV_CRC,NLG5_E_F_CRC,NLG5_E_SDT_CT,NLG5_E_SDT_AH,NLG5_E_SDT_BV,NLG5_E_SDT_BT,NLG5_E_C_RX,NLG5_E_C_TX,NLG5_E_C_VOR,NLG5_E_PL_IT,NLG5_E_PL_BV,NLG5_E_PL_MV
  Data Type Conversion{,1..33} (34 alike) : DataTypeConversion
  Out1 : Outport
  wires:
  Data Type Conversion33/1 -> Bus Creator/34  "NLG5_E_PL_MV"
  Data Type Conversion32/1 -> Bus Creator/33  "NLG5_E_PL_BV"
  Data Type Conversion31/1 -> Bus Creator/32  "NLG5_E_PL_IT"
  Data Type Conversion30/1 -> Bus Creator/31  "NLG5_E_C_VOR"
  Data Type Conversion29/1 -> Bus Creator/30  "NLG5_E_C_TX"
  Data Type Conversion28/1 -> Bus Creator/29  "NLG5_E_C_RX"
  Data Type Conversion27/1 -> Bus Creator/28  "NLG5_E_SDT_BT"
  Data Type Conversion26/1 -> Bus Creator/27  "NLG5_E_SDT_BV"
  Data Type Conversion25/1 -> Bus Creator/26  "NLG5_E_SDT_AH"
  Data Type Conversion24/1 -> Bus Creator/25  "NLG5_E_SDT_CT"
  Data Type Conversion23/1 -> Bus Creator/24  "NLG5_E_F_CRC"
  Data Type Conversion22/1 -> Bus Creator/23  "NLG5_E_NV_CRC"
  Data Type Conversion21/1 -> Bus Creator/22  "NLG5_E_ES_CRC"
  Data Type Conversion20/1 -> Bus Creator/21  "NLG5_E_EP_CRC"
  Data Type Conversion19/1 -> Bus Creator/20  "NLG5_E_WDT"
  Data Type Conversion18/1 -> Bus Creator/19  "NLG5_E_INIT"
  Data Type Conversion17/1 -> Bus Creator/18  "NLG5_E_C_TO"
  Data Type Conversion16/1 -> Bus Creator/17  "NLG5_E_C_OFF"
  Data Type Conversion15/1 -> Bus Creator/16  "NLG5_E_B_P"
  Data Type Conversion14/1 -> Bus Creator/15  "NLG5_E_T_C"
  Data Type Conversion13/1 -> Bus Creator/14  "NLG5_E_T_POW"
  Data Type Conversion12/1 -> Bus Creator/13  "NLG5_E_T_DIO"
  Data Type Conversion10/1 -> Bus Creator/12  "NLG5_E_T_TR"
  Data Type Conversion11/1 -> Bus Creator/11  "NLG5_E_T_EXT1"
  Data Type Conversion9/1 -> Bus Creator/10  "NLG5_E_T_EXT2"
  Data Type Conversion8/1 -> Bus Creator/9  "NLG5_E_T_EXT3"
  Data Type Conversion7/1 -> Bus Creator/8  "NLG5_E_OOV"
  Data Type Conversion6/1 -> Bus Creator/7  "NLG5_E_MOV_I"
  Data Type Conversion5/1 -> Bus Creator/6  "NLG5_E_MOV_II"
  Bus Selector/26 -> Data Type Conversion25/1  "<NLG5_E_SDT_AH>"
  Bus Selector/25 -> Data Type Conversion24/1  "<NLG5_E_SDT_CT>"
  Bus Selector/24 -> Data Type Conversion23/1  "<NLG5_E_F_CRC>"
  Bus Selector/23 -> Data Type Conversion22/1  "<NLG5_E_NV_CRC>"
  Bus Selector/22 -> Data Type Conversion21/1  "<NLG5_E_ES_CRC>"
  Bus Selector/21 -> Data Type Conversion20/1  "<NLG5_E_EP_CRC>"
  Bus Selector/20 -> Data Type Conversion19/1  "<NLG5_E_WDT>"
  Bus Selector/19 -> Data Type Conversion18/1  "<NLG5_E_INIT>"
  Bus Selector/18 -> Data Type Conversion17/1  "<NLG5_E_C_TO>"
  Bus Selector/17 -> Data Type Conversion16/1  "<NLG5_E_C_OFF>"
  Bus Selector/16 -> Data Type Conversion15/1  "<NLG5_E_B_P>"
  Bus Selector/15 -> Data Type Conversion14/1  "<NLG5_E_T_C>"
  Bus Selector/14 -> Data Type Conversion13/1  "<NLG5_E_T_POW>"
  Bus Selector/13 -> Data Type Conversion12/1  "<NLG5_E_T_DIO>"
  Bus Selector/12 -> Data Type Conversion10/1  "<NLG5_E_T_TR>"
  Bus Selector/11 -> Data Type Conversion11/1  "<NLG5_E_T_EXT1>"
  Bus Selector/10 -> Data Type Conversion9/1  "<NLG5_E_T_EXT2>"
  Bus Selector/9 -> Data Type Conversion8/1  "<NLG5_E_T_EXT3>"
  Bus Selector/8 -> Data Type Conversion7/1  "<NLG5_E_OOV>"
  Bus Selector/7 -> Data Type Conversion6/1  "<NLG5_E_MOV_I>"
  Bus Selector/27 -> Data Type Conversion26/1  "<NLG5_E_SDT_BV>"
  Bus Selector/28 -> Data Type Conversion27/1  "<NLG5_E_SDT_BT>"
  Bus Selector/29 -> Data Type Conversion28/1  "<NLG5_E_C_RX>"
  Bus Selector/30 -> Data Type Conversion29/1  "<NLG5_E_C_TX>"
  Bus Selector/31 -> Data Type Conversion30/1  "<NLG5_E_C_VOR>"
  Bus Selector/32 -> Data Type Conversion31/1  "<NLG5_E_PL_IT>"
  Bus Selector/33 -> Data Type Conversion32/1  "<NLG5_E_PL_BV>"
  Bus Selector/34 -> Data Type Conversion33/1  "<NLG5_E_PL_MV>"
  Bus Selector/6 -> Data Type Conversion5/1  "<NLG5_E_MOV_II>"
  Bus Creator/1 -> Out1/1  "NLG5_ERR"
  Data Type Conversion3/1 -> Bus Creator/4  "NLG5_E_P_OM"
  Data Type Conversion2/1 -> Bus Creator/3  "NLG5_E_P_MV"
  Data Type Conversion1/1 -> Bus Creator/2  "NLG5_E_OF"
  Data Type Conversion/1 -> Bus Creator/1  "NLG5_E_MF"
  Bus Selector/4 -> Data Type Conversion3/1  "<NLG5_E_P_OM>"
  Bus Selector/3 -> Data Type Conversion2/1  "<NLG5_E_P_MV>"
  Bus Selector/2 -> Data Type Conversion1/1  "<NLG5_E_OF>"
  Bus Selector/1 -> Data Type Conversion/1  "<NLG5_E_MF>"
  In1/1 -> Bus Selector/1
  Bus Selector/5 -> Data Type Conversion4/1  "<NLG5_E_SC>"
  Data Type Conversion4/1 -> Bus Creator/5  "NLG5_E_SC"

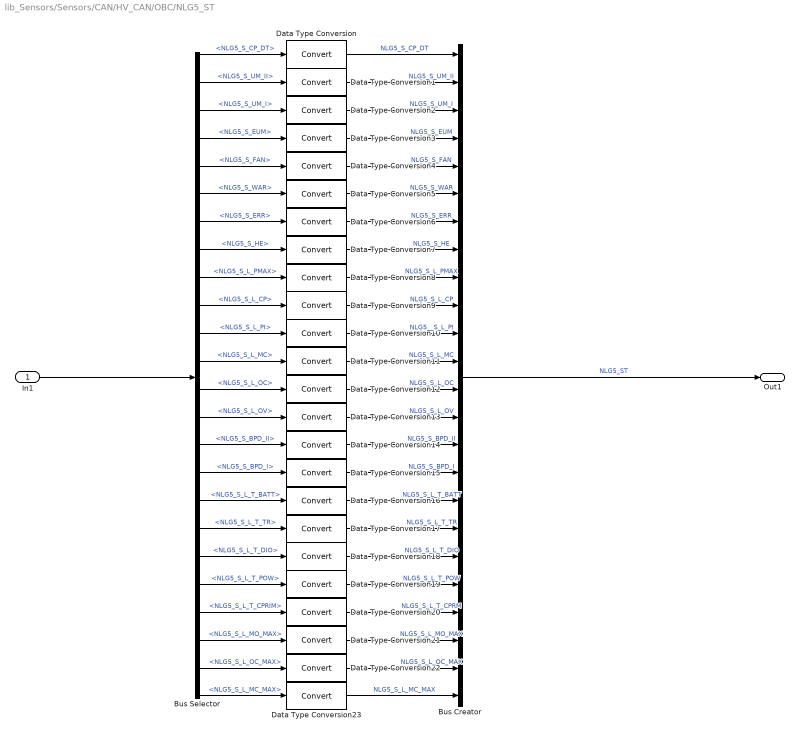
== system lib_Sensors/Sensors/CAN/HV_CAN/OBC/NLG5_ST ==
  In1 : Inport
  Bus Creator : BusCreator  Inputs=24
  Bus Selector : BusSelector  OutputSignals=NLG5_S_CP_DT,NLG5_S_UM_II,NLG5_S_UM_I,NLG5_S_EUM,NLG5_S_FAN,NLG5_S_WAR,NLG5_S_ERR,NLG5_S_HE,NLG5_S_L_PMAX,NLG5_S_L_CP,NLG5_S_L_PI,NLG5_S_L_MC,NLG5_S_L_OC,NLG5_S_L_OV,NLG5_S_BPD_II,NLG5_S_BPD_I,NLG5_S_L_T_BATT,NLG5_S_L_T_TR,NLG5_S_L_T_DIO,NLG5_S_L_T_POW,NLG5_S_L_T_CPRIM,NLG5_S_L_MO_MAX,NLG5_S_L_OC_MAX,NLG5_S_L_MC_MAX
  Data Type Conversion{,1..23} (24 alike) : DataTypeConversion
  Out1 : Outport
  wires:
  Data Type Conversion23/1 -> Bus Creator/24  "NLG5_S_L_MC_MAX"
  Data Type Conversion22/1 -> Bus Creator/23  "NLG5_S_L_OC_MAX"
  Data Type Conversion21/1 -> Bus Creator/22  "NLG5_S_L_MO_MAX"
  Data Type Conversion20/1 -> Bus Creator/21  "NLG5_S_L_T_CPRM"
  Data Type Conversion19/1 -> Bus Creator/20  "NLG5_S_L_T_POW"
  Data Type Conversion18/1 -> Bus Creator/19  "NLG5_S_L_T_DIO"
  Data Type Conversion17/1 -> Bus Creator/18  "NLG5_S_L_T_TR"
  Data Type Conversion16/1 -> Bus Creator/17  "NLG5_S_L_T_BATT"
  Data Type Conversion15/1 -> Bus Creator/16  "NLG5_S_BPD_I"
  Data Type Conversion14/1 -> Bus Creator/15  "NLG5_S_BPD_II"
  Data Type Conversion13/1 -> Bus Creator/14  "NLG5_S_L_OV"
  Data Type Conversion12/1 -> Bus Creator/13  "NLG5_S_L_OC"
  Data Type Conversion11/1 -> Bus Creator/12  "NLG5_S_L_MC"
  Data Type Conversion10/1 -> Bus Creator/11  "NLG5__S_L_PI"
  Data Type Conversion9/1 -> Bus Creator/10  "NLG5_S_L_CP"
  Data Type Conversion8/1 -> Bus Creator/9  "NLG5_S_L_PMAX"
  Data Type Conversion6/1 -> Bus Creator/7  "NLG5_S_ERR"
  Data Type Conversion7/1 -> Bus Creator/8  "NLG5_S_HE"
  Data Type Conversion5/1 -> Bus Creator/6  "NLG5_S_WAR"
  Bus Selector/24 -> Data Type Conversion23/1  "<NLG5_S_L_MC_MAX>"
  Bus Selector/23 -> Data Type Conversion22/1  "<NLG5_S_L_OC_MAX>"
  Bus Selector/22 -> Data Type Conversion21/1  "<NLG5_S_L_MO_MAX>"
  Bus Selector/21 -> Data Type Conversion20/1  "<NLG5_S_L_T_CPRIM>"
  Bus Selector/20 -> Data Type Conversion19/1  "<NLG5_S_L_T_POW>"
  Bus Selector/19 -> Data Type Conversion18/1  "<NLG5_S_L_T_DIO>"
  Bus Selector/18 -> Data Type Conversion17/1  "<NLG5_S_L_T_TR>"
  Bus Selector/17 -> Data Type Conversion16/1  "<NLG5_S_L_T_BATT>"
  Bus Selector/16 -> Data Type Conversion15/1  "<NLG5_S_BPD_I>"
  Bus Selector/15 -> Data Type Conversion14/1  "<NLG5_S_BPD_II>"
  Bus Selector/14 -> Data Type Conversion13/1  "<NLG5_S_L_OV>"
  Bus Selector/13 -> Data Type Conversion12/1  "<NLG5_S_L_OC>"
  Bus Selector/12 -> Data Type Conversion11/1  "<NLG5_S_L_MC>"
  Bus Selector/11 -> Data Type Conversion10/1  "<NLG5_S_L_PI>"
  Bus Selector/10 -> Data Type Conversion9/1  "<NLG5_S_L_CP>"
  Bus Selector/9 -> Data Type Conversion8/1  "<NLG5_S_L_PMAX>"
  Bus Selector/8 -> Data Type Conversion7/1  "<NLG5_S_HE>"
  Bus Selector/7 -> Data Type Conversion6/1  "<NLG5_S_ERR>"
  Bus Selector/6 -> Data Type Conversion5/1  "<NLG5_S_WAR>"
  Bus Creator/1 -> Out1/1  "NLG5_ST"
  Data Type Conversion3/1 -> Bus Creator/4  "NLG5_S_EUM"
  Data Type Conversion2/1 -> Bus Creator/3  "NLG5_S_UM_I"
  Data Type Conversion1/1 -> Bus Creator/2  "NLG5_S_UM_II"
  Data Type Conversion/1 -> Bus Creator/1  "NLG5_S_CP_DT"
  Bus Selector/4 -> Data Type Conversion3/1  "<NLG5_S_EUM>"
  Bus Selector/3 -> Data Type Conversion2/1  "<NLG5_S_UM_I>"
  Bus Selector/2 -> Data Type Conversion1/1  "<NLG5_S_UM_II>"
  Bus Selector/1 -> Data Type Conversion/1  "<NLG5_S_CP_DT>"
  In1/1 -> Bus Selector/1
  Bus Selector/5 -> Data Type Conversion4/1  "<NLG5_S_FAN>"
  Data Type Conversion4/1 -> Bus Creator/5  "NLG5_S_FAN"

== system lib_Sensors/Sensors/CAN/HV_CAN/OBC/NLG5_TEMP ==
  In1 : Inport
  Bus Creator : BusCreator  Inputs=4
  Bus Selector : BusSelector  OutputSignals=NLG5_P_TMP,NLG5_TMP_EXT1,NLG5_TMP_EXT2,NLG5_TMP_EXT3
  Data Type Conversion{,1..3} (4 alike) : DataTypeConversion
  Out1 : Outport
  wires:
  Bus Creator/1 -> Out1/1  "NLG5_TEMP"
  Data Type Conversion3/1 -> Bus Creator/4  "NLG5_TMP_EXT3"
  Data Type Conversion2/1 -> Bus Creator/3  "NLG5_TMP_EXT2"
  Data Type Conversion1/1 -> Bus Creator/2  "NLG5_TMP_EXT1"
  Data Type Conversion/1 -> Bus Creator/1  "NLG5_P_TMP"
  Bus Selector/4 -> Data Type Conversion3/1  "<NLG5_TMP_EXT3>"
  Bus Selector/3 -> Data Type Conversion2/1  "<NLG5_TMP_EXT2>"
  Bus Selector/2 -> Data Type Conversion1/1  "<NLG5_TMP_EXT1>"
  Bus Selector/1 -> Data Type Conversion/1  "<NLG5_P_TMP>"
  In1/1 -> Bus Selector/1

== system lib_Sensors/Sensors/CAN/VEH_CAN/BCM/PPEI_Brake_Apply_Status ==
  In1 : Inport
  Out1 : Outport
  wires:
  In1/1 -> Out1/1  "BrkPdlPos"

== system lib_Sensors/Sensors/CAN/VEH_CAN/BCM/PPEI_Platfrom_General_Status ==
  In1 : Inport
  Out1 : Outport
  wires:
  In1/1 -> Out1/1  "SysPwrMd"

== system lib_Sensors/Sensors/CAN/VEH_CAN/EBCM/PPEI_Chassis_General_Status_1 ==
  In1 : Inport
  Out1 : Outport
  wires:
  In1/1 -> Out1/1  "BrkPdlDrvAppPrsDetcd"
